simulink model "flightController"  (R2023b)
settings: Solver=ode3  StartTime=0  StopTime=TFinal  FixedStep=Ts  RelTol=1e-3  EnableMultiTasking=on
undefined symbols (not defined in the file): Controller, DiscIntNeverNeededParam, g, PD, PI, PID, Ts, Vehicle
libraries: simulink x7, slpidlib x3, rllib x2, dspstat3 x2, fuzblock x2
(part 2 of 2)

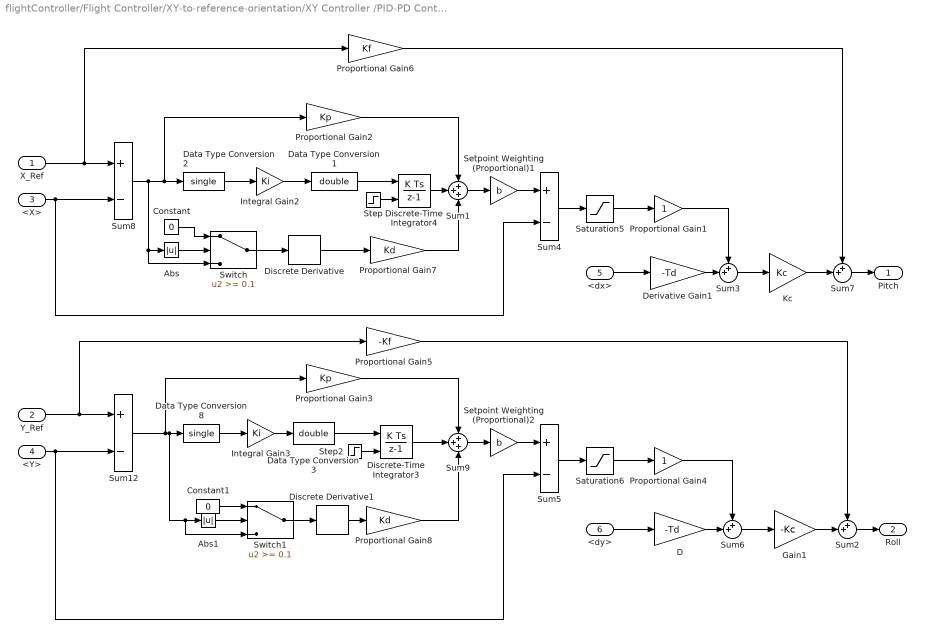
== system flightController/Flight Controller/XY-to-reference-orientation/XY Controller /PID-PD Controller  ==
  X_Ref : Inport
  Y_Ref : Inport  Port=2
  <X> : Inport  Port=3
  <Y> : Inport  Port=4
  <dx> : Inport  Port=5
  <dy> : Inport  Port=6
  Abs : Abs  SaturateOnIntegerOverflow=off
  Abs1 : Abs  SaturateOnIntegerOverflow=off
  Constant : Constant  Value=0  SampleTime=-1
  Constant1 : Constant  Value=0  SampleTime=-1
  D : Gain  Gain=-Td
  Data Type Conversion1 : DataTypeConversion  OutDataTypeStr=double  SaturateOnIntegerOverflow=off  RndMeth=Floor
  Data Type Conversion2 : DataTypeConversion  OutDataTypeStr=single  SaturateOnIntegerOverflow=off  RndMeth=Floor
  Data Type Conversion3 : DataTypeConversion  OutDataTypeStr=double  SaturateOnIntegerOverflow=off  RndMeth=Floor
  Data Type Conversion8 : DataTypeConversion  OutDataTypeStr=single  SaturateOnIntegerOverflow=off  RndMeth=Floor
  Derivative Gain1 : Gain  DisableCoverage=on  Gain=-Td
  Discrete Derivative : simulink/Discrete/Discrete Derivative  gainval=1.0  ICPrevScaledInput=0.0  OutMin=[]  OutMax=[]  OutDataType=fixdt(1, 16)  OutScaling=2^-10  DoSatur=off
  Discrete Derivative1 : simulink/Discrete/Discrete Derivative  gainval=1.0  ICPrevScaledInput=0.0  OutMin=[]  OutMax=[]  OutDataType=fixdt(1, 16)  OutScaling=2^-10  DoSatur=off
  Discrete-Time Integrator3 : DiscreteIntegrator  ExternalReset=falling  SampleTime=Ts  ICPrevOutput=DiscIntNeverNeededParam  ICPrevScaledInput=DiscIntNeverNeededParam
  Discrete-Time Integrator4 : DiscreteIntegrator  ExternalReset=falling  SampleTime=Ts  ICPrevOutput=DiscIntNeverNeededParam  ICPrevScaledInput=DiscIntNeverNeededParam
  Gain1 : Gain  Gain=-Kc
  Integral Gain2 : Gain  DisableCoverage=on  Gain=Ki
  Integral Gain3 : Gain  DisableCoverage=on  Gain=Ki
  Kc : Gain  Gain=Kc
  Proportional Gain1 : Gain
  Proportional Gain2 : Gain  Gain=Kp
  Proportional Gain3 : Gain  Gain=Kp
  Proportional Gain4 : Gain
  Proportional Gain5 : Gain  Gain=-Kf
  Proportional Gain6 : Gain  Gain=Kf
  Proportional Gain7 : Gain  Gain=Kd
  Proportional Gain8 : Gain  Gain=Kd
  Saturation5 : Saturate  UpperLimit=3  LowerLimit=-3  OutDataTypeStr=single
  Saturation6 : Saturate  UpperLimit=3  LowerLimit=-3  OutDataTypeStr=single
  Setpoint Weighting (Proportional)1 : Gain  DisableCoverage=on  Gain=b
  Setpoint Weighting (Proportional)2 : Gain  DisableCoverage=on  Gain=b
  Step : Step  Time=49  Before=1  After=0  SampleTime=Ts
  Step2 : Step  Time=49  Before=1  After=0  SampleTime=Ts
  Sum1 : Sum  Inputs=+++
  Sum{4..5,8,12} (4 alike) : Sum  DisableCoverage=on  Inputs=+-
  Sum{2..3,6..7} (4 alike) : Sum  Inputs=++|
  Sum9 : Sum  Inputs=+++
  Switch : Switch  Threshold=0.1  SaturateOnIntegerOverflow=off  InputSameDT=off
  Switch1 : Switch  Threshold=0.1  SaturateOnIntegerOverflow=off  InputSameDT=off
  Pitch : Outport  OutDataTypeStr=single  VectorParamsAs1DForOutWhenUnconnected=off
  Roll : Outport  Port=2  OutDataTypeStr=single  VectorParamsAs1DForOutWhenUnconnected=off
  wires:
  X_Ref/1 -> Proportional Gain6/1, Sum8/1
  Proportional Gain6/1 -> Sum7/1
  Proportional Gain5/1 -> Sum2/1
  Sum4/1 -> Saturation5/1
  Sum1/1 -> Setpoint Weighting (Proportional)1/1
  Saturation5/1 -> Proportional Gain1/1
  <Y>/1 -> Sum12/2, Sum5/2
  Sum6/1 -> Gain1/1
  <X>/1 -> Sum8/2, Sum4/2
  Sum3/1 -> Kc/1
  Setpoint Weighting (Proportional)1/1 -> Sum4/1
  Proportional Gain1/1 -> Sum3/1
  Derivative Gain1/1 -> Sum3/2
  <dy>/1 -> D/1
  <dx>/1 -> Derivative Gain1/1
  Gain1/1 -> Sum2/2
  Kc/1 -> Sum7/2
  Proportional Gain2/1 -> Sum1/1
  Data Type Conversion1/1 -> Discrete-Time Integrator4/1
  Integral Gain2/1 -> Data Type Conversion1/1
  Discrete-Time Integrator4/1 -> Sum1/2
  Data Type Conversion2/1 -> Integral Gain2/1
  Sum8/1 -> Switch/3, Abs/1, Data Type Conversion2/1, Proportional Gain2/1
  Data Type Conversion8/1 -> Integral Gain3/1
  Discrete-Time Integrator3/1 -> Sum9/2
  Integral Gain3/1 -> Data Type Conversion3/1
  Y_Ref/1 -> Sum12/1, Proportional Gain5/1
  Data Type Conversion3/1 -> Discrete-Time Integrator3/1
  Proportional Gain3/1 -> Sum9/1
  Step/1 -> Discrete-Time Integrator4/2
  Step2/1 -> Discrete-Time Integrator3/2
  Setpoint Weighting (Proportional)2/1 -> Sum5/1
  Saturation6/1 -> Proportional Gain4/1
  Sum9/1 -> Setpoint Weighting (Proportional)2/1
  Sum5/1 -> Saturation6/1
  D/1 -> Sum6/2
  Proportional Gain4/1 -> Sum6/1
  Proportional Gain7/1 -> Sum1/3
  Constant/1 -> Switch/1
  Switch/1 -> Discrete Derivative/1
  Abs/1 -> Switch/2
  Abs1/1 -> Switch1/2
  Switch1/1 -> Discrete Derivative1/1
  Constant1/1 -> Switch1/1
  Proportional Gain8/1 -> Sum9/3
  Sum12/1 -> Abs1/1, Switch1/3, Data Type Conversion8/1, Proportional Gain3/1
  Discrete Derivative/1 -> Proportional Gain7/1
  Discrete Derivative1/1 -> Proportional Gain8/1
  Sum2/1 -> Roll/1
  Sum7/1 -> Pitch/1

== system flightController/Flight Controller/Yaw/Yaw RL Agent/observations ==
  In1 : Inport
  Bus Selector : BusSelector  OutputSignals=X,Y,Z,yaw,pitch,roll,dx,dy,dz,p,q,r
  Bus Selector1 : BusSelector  OutputSignals=yaw
  Mux : Mux  Inputs=12
  Out1 : Outport
  yaw : Outport  Port=2
  wires:
  In1/1 -> Bus Selector1/1, Bus Selector/1
  Bus Selector/1 -> Mux/1  "<X>"
  Bus Selector/2 -> Mux/2  "<Y>"
  Bus Selector/3 -> Mux/3  "<Z>"
  Bus Selector/4 -> Mux/4  "<yaw>"
  Bus Selector/5 -> Mux/5  "<pitch>"
  Bus Selector/6 -> Mux/6  "<roll>"
  Bus Selector/7 -> Mux/7  "<dx>"
  Bus Selector/8 -> Mux/8  "<dy>"
  Bus Selector/9 -> Mux/9  "<dz>"
  Bus Selector/10 -> Mux/10  "<p>"
  Bus Selector/11 -> Mux/11  "<q>"
  Bus Selector/12 -> Mux/12  "<r>"
  Mux/1 -> Out1/1
  Bus Selector1/1 -> yaw/1  "<yaw>"

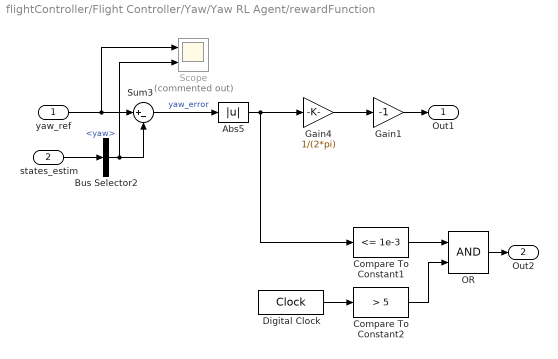
== system flightController/Flight Controller/Yaw/Yaw RL Agent/rewardFunction ==
  yaw_ref : Inport
  states_estim : Inport  Port=2
  Abs5 : Abs  SaturateOnIntegerOverflow=off
  Bus Selector2 : BusSelector  OutputSignals=yaw
  Compare To Constant1 : simulink/Logic and Bit Operations/Compare To Constant  relop=<=  const=1e-3  OutDataTypeStr=boolean
  Compare To Constant2 : simulink/Logic and Bit Operations/Compare To Constant  relop=>  const=5  OutDataTypeStr=boolean
  Digital Clock : DigitalClock  SampleTime=Ts
  Gain1 : Gain  Gain=-1
  Gain4 : Gain  Gain=1/(2*pi)
  OR : Logic  AllPortsSameDT=off  OutDataTypeStr=boolean
  Scope : Scope  Commented=on  NumInputPorts=2
  Sum3 : Sum  Inputs=|+-
  Out1 : Outport
  Out2 : Outport  Port=2
  wires:
  Gain1/1 -> Out1/1
  states_estim/1 -> Bus Selector2/1
  Sum3/1 -> Abs5/1  "yaw_error"
  Abs5/1 -> Compare To Constant1/1, Gain4/1
  Gain4/1 -> Gain1/1
  OR/1 -> Out2/1
  Digital Clock/1 -> Compare To Constant2/1
  yaw_ref/1 -> Sum3/1, Scope/1
  Bus Selector2/1 -> Scope/2, Sum3/2  "<yaw>"
  Compare To Constant1/1 -> OR/1
  Compare To Constant2/1 -> OR/2

== system flightController/Flight Controller/gravity feedforward//equilibrium thrust/Z Controller Subsystem/PD Controller  ==
  PosZ : Inport
  <Z> : Inport  Port=2
  <dz> : Inport  Port=3
  Derivative Gain : Gain  DisableCoverage=on  Gain=-Td
  Kc : Gain  Gain=Kc
  Proportional Gain : Gain
  Setpoint Weighting (Proportional) : Gain  DisableCoverage=on  Gain=b
  Sum3 : Sum  Inputs=|++
  Sum4 : Sum  DisableCoverage=on  Inputs=+-
  Altitude : Outport  VectorParamsAs1DForOutWhenUnconnected=off
  wires:
  Kc/1 -> Altitude/1
  <dz>/1 -> Derivative Gain/1
  Derivative Gain/1 -> Sum3/2
  Proportional Gain/1 -> Sum3/1
  Setpoint Weighting (Proportional)/1 -> Sum4/1
  Sum3/1 -> Kc/1
  <Z>/1 -> Sum4/2
  Sum4/1 -> Proportional Gain/1
  PosZ/1 -> Setpoint Weighting (Proportional)/1

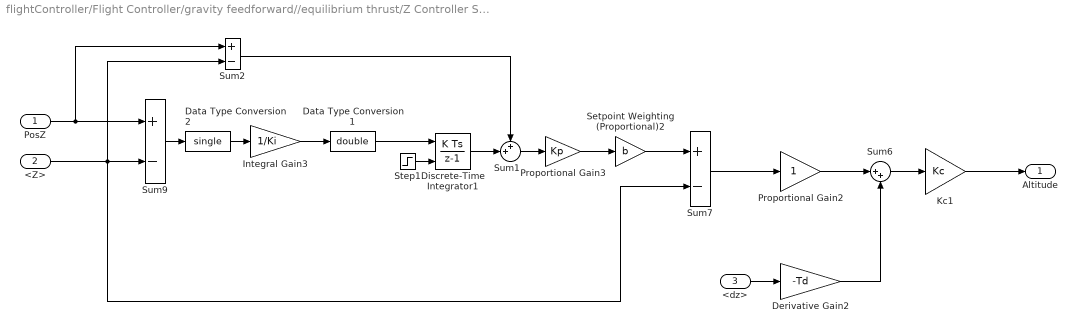
== system flightController/Flight Controller/gravity feedforward//equilibrium thrust/Z Controller Subsystem/PI-PD Controller  ==
  PosZ : Inport
  <Z> : Inport  Port=2
  <dz> : Inport  Port=3
  Data Type Conversion1 : DataTypeConversion  OutDataTypeStr=double  SaturateOnIntegerOverflow=off  RndMeth=Floor
  Data Type Conversion2 : DataTypeConversion  OutDataTypeStr=single  SaturateOnIntegerOverflow=off  RndMeth=Floor
  Derivative Gain2 : Gain  DisableCoverage=on  Gain=-Td
  Discrete-Time Integrator1 : DiscreteIntegrator  ExternalReset=falling  SampleTime=Ts  ICPrevOutput=DiscIntNeverNeededParam  ICPrevScaledInput=DiscIntNeverNeededParam
  Integral Gain3 : Gain  DisableCoverage=on  Gain=1/Ki
  Kc1 : Gain  Gain=Kc
  Proportional Gain2 : Gain
  Proportional Gain3 : Gain  Gain=Kp
  Setpoint Weighting (Proportional)2 : Gain  DisableCoverage=on  Gain=b
  Step1 : Step  Time=49  Before=1  After=0  SampleTime=Ts
  Sum1 : Sum  Inputs=++|
  Sum2 : Sum  DisableCoverage=on  Inputs=+-
  Sum6 : Sum  Inputs=|++
  Sum7 : Sum  DisableCoverage=on  Inputs=+-
  Sum9 : Sum  DisableCoverage=on  Inputs=+-
  Altitude : Outport  VectorParamsAs1DForOutWhenUnconnected=off
  wires:
  Setpoint Weighting (Proportional)2/1 -> Sum7/1
  Sum9/1 -> Data Type Conversion2/1
  <Z>/1 -> Sum7/2, Sum9/2, Sum2/2
  Data Type Conversion2/1 -> Integral Gain3/1
  Discrete-Time Integrator1/1 -> Sum1/2
  Sum7/1 -> Proportional Gain2/1
  Integral Gain3/1 -> Data Type Conversion1/1
  Sum2/1 -> Sum1/1
  PosZ/1 -> Sum2/1, Sum9/1
  Data Type Conversion1/1 -> Discrete-Time Integrator1/1
  Proportional Gain2/1 -> Sum6/1
  Derivative Gain2/1 -> Sum6/2
  Sum6/1 -> Kc1/1
  <dz>/1 -> Derivative Gain2/1
  Sum1/1 -> Proportional Gain3/1
  Kc1/1 -> Altitude/1
  Proportional Gain3/1 -> Setpoint Weighting (Proportional)2/1
  Step1/1 -> Discrete-Time Integrator1/2

== matlab function flightController/Flight Controller/Attitude/Roll & Pitch RL Agent/rewardFunction/MATLAB Function ==
  data: u input; y output
function y = WrapPi(u)

u2 = mod(u,2*pi);

if u2 > pi
    y = u2 - 2*pi;
elseif u2 < -pi
    y = u2 + 2*pi;
else
    y = u2;
end

== matlab function flightController/Flight Controller/Attitude/Roll & Pitch RL Agent/rewardFunction/MATLAB Function1 ==
  data: u input; y output
function y = WrapPi(u)

u2 = mod(u,2*pi);

if u2 > pi
    y = u2 - 2*pi;
elseif u2 < -pi
    y = u2 + 2*pi;
else
    y = u2;
end
